simulink model "Ecotron"  (R2019b)
settings: Solver=FixedStepAuto  StartTime=0.0  StopTime=1  FixedStep=0.001  RelTol=1e-3  EnableMultiTasking=on
InitFcn:
  | EcoCoder_PreCheckLic();
libraries: CoderSF_BSW_Libs x228, SF_CanService_Libs x49, simulink x33, dspstat3 x6
(part 6 of 6)

== system Ecotron/Main /LongControl /ACC Control/Long PID/Acceleration ==
  speed : Inport
  Moving Average1 : dspstat3/Moving Average  Method=Sliding window  ForgettingFactorPort=off  SpecifyWindowLength=on  WindowLength=100  ForgettingFactor=0.9  SimulateUsing=Code generation
  Moving Average2 : dspstat3/Moving Average  Method=Sliding window  ForgettingFactorPort=off  SpecifyWindowLength=on  WindowLength=100  ForgettingFactor=0.9  SimulateUsing=Code generation
  Write Measurement : CoderSF_BSW_Libs/Calibration & Measurement/Write Measurement  variable_name=Golf_ACC  variable_value=0  variable_type=single  numD=1  unitStr=""  descStr=""
      settings: AttributesFormatString=type:%<variable_type> Dimensions:%<numD>  SourceProductName=EcoCoder Blocks
  Write Measurement1 : CoderSF_BSW_Libs/Calibration & Measurement/Write Measurement  variable_name=debug_Golf_speed  variable_value=0  variable_type=single  numD=1  unitStr=ms  descStr=""
      settings: AttributesFormatString=type:%<variable_type> Dimensions:%<numD>  SourceProductName=EcoCoder Blocks
  Write Measurement2 : CoderSF_BSW_Libs/Calibration & Measurement/Write Measurement  variable_name=debug_Golf_speed_movAvg  variable_value=0  variable_type=single  numD=1  unitStr=ms  descStr=""
      settings: AttributesFormatString=type:%<variable_type> Dimensions:%<numD>  SourceProductName=EcoCoder Blocks
  Write Measurement3 : CoderSF_BSW_Libs/Calibration & Measurement/Write Measurement  variable_name=debug_Golf_ACC  variable_value=0  variable_type=single  numD=1  unitStr=ms2  descStr=""
      settings: AttributesFormatString=type:%<variable_type> Dimensions:%<numD>  SourceProductName=EcoCoder Blocks
  basic derivative1 : Subsystem
  m/s^2 : Outport
  wires:
  Moving Average1/1 -> Write Measurement2/1, basic derivative1/1(In1)  "m/s"
  speed/1 -> Write Measurement1/1, Moving Average1/1
  basic derivative1/1(Out1) -> Write Measurement3/1, Moving Average2/1
  Moving Average2/1 -> Write Measurement/1, m/s^2/1  "m/s^2"

== system Ecotron/Main /LongControl /ACC Control/Long PID/Acceleration1 ==
  speed : Inport
  Moving Average1 : dspstat3/Moving Average  Method=Sliding window  ForgettingFactorPort=off  SpecifyWindowLength=on  WindowLength=200  ForgettingFactor=0.9  SimulateUsing=Code generation
  Moving Average2 : dspstat3/Moving Average  Method=Sliding window  ForgettingFactorPort=off  SpecifyWindowLength=on  WindowLength=200  ForgettingFactor=0.9  SimulateUsing=Code generation
  Write Measurement : CoderSF_BSW_Libs/Calibration & Measurement/Write Measurement  variable_name=Golf_ACC_200sample  variable_value=0  variable_type=single  numD=1  unitStr=""  descStr=""
      settings: AttributesFormatString=type:%<variable_type> Dimensions:%<numD>  SourceProductName=EcoCoder Blocks
  Write Measurement2 : CoderSF_BSW_Libs/Calibration & Measurement/Write Measurement  variable_name=debug_Golf_speed_movAvg150sample  variable_value=0  variable_type=single  numD=1  unitStr=ms  descStr=""
      settings: AttributesFormatString=type:%<variable_type> Dimensions:%<numD>  SourceProductName=EcoCoder Blocks
  Write Measurement3 : CoderSF_BSW_Libs/Calibration & Measurement/Write Measurement  variable_name=debug_Golf_ACC150sample  variable_value=0  variable_type=single  numD=1  unitStr=ms2  descStr=""
      settings: AttributesFormatString=type:%<variable_type> Dimensions:%<numD>  SourceProductName=EcoCoder Blocks
  basic derivative1 : Subsystem
  m/s^2 : Outport
  wires:
  Moving Average2/1 -> m/s^2/1, Write Measurement/1  "m/s^2"
  basic derivative1/1(Out1) -> Moving Average2/1, Write Measurement3/1
  speed/1 -> Moving Average1/1
  Moving Average1/1 -> basic derivative1/1(In1), Write Measurement2/1  "m/s"

== system Ecotron/Main /LongControl /ACC Control/Long PID/CascadedPID ==
  AccCMD : Inport
  m/s^2 : Inport  Port=2
  Motor torque : Inport  Port=3
  Gear : Inport  Port=4
  "Reset " : Inport  Port=5
  1-D Lookup Table : Lookup_n-D  NumberOfTableDimensions=1  BreakpointsForDimension1=[0:5]  Table=[0 118 194 291 390 516]  InternalRulePriority=Speed  RndMeth=Simplest  InputSameDT=on
  Multiply : Gain  Gain=0.01
  PID Controller : simulink/Continuous/PID Controller  Controller=PID  Form=Parallel  TimeDomain=Discrete-time  SampleTime=1/100  IntegratorMethod=Forward Euler  FilterMethod=Forward Euler  ControllerParametersSource=external  P=1  I=1  D=0  UseFilter=off  N=100  TunerSelectOption=Transfer Function Based (PID Tuner App)  InitialConditionSource=internal  InitialConditionForIntegrator=0  InitialConditionForFilter=0  DifferentiatorICPrevScaledInput=0  ExternalReset=either  TrackingMode=off  Kt=1  LimitOutput=on  UpperSaturationLimit=120  LowerSaturationLimit=0  LinearizeAsGain=on  AntiWindupMode=clamping  Kb=1  POutMin=[]  POutMax=[]  IOutMin=[]  IOutMax=[]  DOutMin=[]  DOutMax=[]  NOutMin=[]  NOutMax=[]  SumOutMin=[]  SumOutMax=[]  SaturationOutMin=[]  SaturationOutMax=[]  PParamMin=[]  PParamMax=[]  IParamMin=[]  IParamMax=[]  DParamMin=[]  DParamMax=[]  NParamMin=[]  NParamMax=[]  KbParamMin=[]  KbParamMax=[]  KtParamMin=[]  KtParamMax=[]  KbOutMin=[]  KbOutMax=[]  KtOutMin=[]  KtOutMax=[]  IntegratorOutMin=[]  IntegratorOutMax=[]  FilterOutMin=[]  FilterOutMax=[]  SumI1OutMin=[]  SumI1OutMax=[]  SumI2OutMin=[]  SumI2OutMax=[]  SumI3OutMin=[]  SumI3OutMax=[]  SumI4OutMin=[]  SumI4OutMax=[]  SumDOutMin=[]  SumDOutMax=[]  DifferentiatorOutMin=[]  DifferentiatorOutMax=[]  FilterDiffOutCoefMin=[]  FilterDiffOutCoefMax=[]  ReciprocalOutMin=[]  ReciprocalOutMax=[]  SumDenOutMin=[]  SumDenOutMax=[]  SumNumOutMin=[]  SumNumOutMax=[]  DivideOutMin=[]  DivideOutMax=[]  IntegratorContinuousStateAttributes=''  IntegratorStateMustResolveToSignalObject=off  IntegratorRTWStateStorageClass=Auto  FilterContinuousStateAttributes=''  FilterStateMustResolveToSignalObject=off  FilterRTWStateStorageClass=Auto  ParallelPVariant=ExternalParameters  IdealPVariant=Disabled  IVariant=ExternalParameters  DVariant=ExternalParameters  IntegratorVariant=Discrete  SatVariant=Enabled  AWVariant=DiscClampingParallel  PCopyVariant=Disabled  TRVariant=Disabled  FdbkBlocksVariant=Forward  IdealPFdbkVariant=Disabled  SatFdbkVariant=Disabled  DerivativeFilterVariant=Differentiator  NVariant=Passthrough  NCopyVariant=Disabled_SignalSpec  FilterICVariant=InternalICsDifferentiator  IntegratorICVariant=InternalICs  ExternalResetVariant=ExternalReset  TRSumVariant=Passthrough  SumFdbkVariant=Disabled  SumVariant=Sum_PID
  PID Controller1 : simulink/Continuous/PID Controller  Controller=PID  Form=Parallel  TimeDomain=Discrete-time  SampleTime=1/100  IntegratorMethod=Forward Euler  FilterMethod=Forward Euler  ControllerParametersSource=external  P=1  I=1  D=0  UseFilter=off  N=100  TunerSelectOption=Transfer Function Based (PID Tuner App)  InitialConditionSource=internal  InitialConditionForIntegrator=0  InitialConditionForFilter=0  DifferentiatorICPrevScaledInput=0  ExternalReset=either  TrackingMode=off  Kt=1  LimitOutput=on  UpperSaturationLimit=50  LowerSaturationLimit=0  LinearizeAsGain=on  AntiWindupMode=clamping  Kb=1  POutMin=[]  POutMax=[]  IOutMin=[]  IOutMax=[]  DOutMin=[]  DOutMax=[]  NOutMin=[]  NOutMax=[]  SumOutMin=[]  SumOutMax=[]  SaturationOutMin=[]  SaturationOutMax=[]  PParamMin=[]  PParamMax=[]  IParamMin=[]  IParamMax=[]  DParamMin=[]  DParamMax=[]  NParamMin=[]  NParamMax=[]  KbParamMin=[]  KbParamMax=[]  KtParamMin=[]  KtParamMax=[]  KbOutMin=[]  KbOutMax=[]  KtOutMin=[]  KtOutMax=[]  IntegratorOutMin=[]  IntegratorOutMax=[]  FilterOutMin=[]  FilterOutMax=[]  SumI1OutMin=[]  SumI1OutMax=[]  SumI2OutMin=[]  SumI2OutMax=[]  SumI3OutMin=[]  SumI3OutMax=[]  SumI4OutMin=[]  SumI4OutMax=[]  SumDOutMin=[]  SumDOutMax=[]  DifferentiatorOutMin=[]  DifferentiatorOutMax=[]  FilterDiffOutCoefMin=[]  FilterDiffOutCoefMax=[]  ReciprocalOutMin=[]  ReciprocalOutMax=[]  SumDenOutMin=[]  SumDenOutMax=[]  SumNumOutMin=[]  SumNumOutMax=[]  DivideOutMin=[]  DivideOutMax=[]  IntegratorContinuousStateAttributes=''  IntegratorStateMustResolveToSignalObject=off  IntegratorRTWStateStorageClass=Auto  FilterContinuousStateAttributes=''  FilterStateMustResolveToSignalObject=off  FilterRTWStateStorageClass=Auto  ParallelPVariant=ExternalParameters  IdealPVariant=Disabled  IVariant=ExternalParameters  DVariant=ExternalParameters  IntegratorVariant=Discrete  SatVariant=Enabled  AWVariant=DiscClampingParallel  PCopyVariant=Disabled  TRVariant=Disabled  FdbkBlocksVariant=Forward  IdealPFdbkVariant=Disabled  SatFdbkVariant=Disabled  DerivativeFilterVariant=Differentiator  NVariant=Passthrough  NCopyVariant=Disabled_SignalSpec  FilterICVariant=InternalICsDifferentiator  IntegratorICVariant=InternalICs  ExternalResetVariant=ExternalReset  TRSumVariant=Passthrough  SumFdbkVariant=Disabled  SumVariant=Sum_PID
  Product : Product
  Product1 : Product
  Read Calibration : CoderSF_BSW_Libs/Calibration & Measurement/Read Calibration  variable_name=Torque_PID_P  variable_value=0.15  variable_type=single  variable_min=[]  variable_max=[]  unitStr=""  descStr=""
      settings: AttributesFormatString=value:%<variable_value> type:%<variable_type> max:%<variable_max> Min:%<variable_min>  SourceProductName=EcoCoder Blocks
  Read Calibration1 : CoderSF_BSW_Libs/Calibration & Measurement/Read Calibration  variable_name=Torque_PID_I  variable_value=0.5  variable_type=single  variable_min=[]  variable_max=[]  unitStr=""  descStr=""
      settings: AttributesFormatString=value:%<variable_value> type:%<variable_type> max:%<variable_max> Min:%<variable_min>  SourceProductName=EcoCoder Blocks
  Read Calibration2 : CoderSF_BSW_Libs/Calibration & Measurement/Read Calibration  variable_name=Torque_PID_D  variable_value=0  variable_type=single  variable_min=[]  variable_max=[]  unitStr=""  descStr=""
      settings: AttributesFormatString=value:%<variable_value> type:%<variable_type> max:%<variable_max> Min:%<variable_min>  SourceProductName=EcoCoder Blocks
  Read Calibration3 : CoderSF_BSW_Libs/Calibration & Measurement/Read Calibration  variable_name=ACC_PID_P  variable_value=0.1  variable_type=single  variable_min=[]  variable_max=[]  unitStr=""  descStr=""
      settings: AttributesFormatString=value:%<variable_value> type:%<variable_type> max:%<variable_max> Min:%<variable_min>  SourceProductName=EcoCoder Blocks
  Read Calibration4 : CoderSF_BSW_Libs/Calibration & Measurement/Read Calibration  variable_name=ACC_PID_I  variable_value=0.4  variable_type=single  variable_min=[]  variable_max=[]  unitStr=""  descStr=""
      settings: AttributesFormatString=value:%<variable_value> type:%<variable_type> max:%<variable_max> Min:%<variable_min>  SourceProductName=EcoCoder Blocks
  Read Calibration5 : CoderSF_BSW_Libs/Calibration & Measurement/Read Calibration  variable_name=ACC_PID_D  variable_value=0  variable_type=single  variable_min=[]  variable_max=[]  unitStr=""  descStr=""
      settings: AttributesFormatString=value:%<variable_value> type:%<variable_type> max:%<variable_max> Min:%<variable_min>  SourceProductName=EcoCoder Blocks
  Subtract : Sum  Inputs=+-
  Subtract1 : Sum  Inputs=+-
  Write Measurement : CoderSF_BSW_Libs/Calibration & Measurement/Write Measurement  variable_name=Motor_requested_Torque  variable_value=0  variable_type=single  numD=1  unitStr=""  descStr=""
      settings: AttributesFormatString=type:%<variable_type> Dimensions:%<numD>  SourceProductName=EcoCoder Blocks
  Gas : Outport
  wires:
  AccCMD/1 -> Subtract/1
  m/s^2/1 -> Subtract/2
  Subtract/1 -> PID Controller/1
  Read Calibration/1 -> PID Controller1/2
  Read Calibration1/1 -> PID Controller1/3
  Read Calibration2/1 -> PID Controller1/4
  Gear/1 -> 1-D Lookup Table/1
  Read Calibration3/1 -> Product/1
  1-D Lookup Table/1 -> Product1/1, Product/2
  Read Calibration4/1 -> Product1/2
  Product/1 -> PID Controller/2
  Product1/1 -> PID Controller/3
  Read Calibration5/1 -> PID Controller/4
  Subtract1/1 -> PID Controller1/1
  PID Controller/1 -> Write Measurement/1, Subtract1/1  "Requested Torque"
  Motor torque/1 -> Subtract1/2
  PID Controller1/1 -> Multiply/1
  Multiply/1 -> Gas/1
  "Reset "/1 -> PID Controller1/5, PID Controller/5

== system Ecotron/Main /LongControl /ACC Control/Long PID/Level converter ==
  Pi in : Inport
  StopMode : Inport  Port=2
  Constant : Constant  Value=50  OutDataTypeStr=single
  Constant1 : Constant  Value=0  OutDataTypeStr=single
  Gain : Gain  Gain=-1
  Gain2 : Gain  Gain=120
  Gain4 : Gain  Gain=100
  Saturation : Saturate  UpperLimit=1  LowerLimit=0
  Saturation1 : Saturate  UpperLimit=1  LowerLimit=0
  Switch : Switch  Criteria=u2 > Threshold
  Switch1 : Switch  Criteria=u2 > Threshold
  Gas : Outport
  Brake : Outport  Port=2
  wires:
  Pi in/1 -> Gain/1, Saturation/1
  Saturation/1 -> Gain4/1  "gas"
  Gain/1 -> Saturation1/1
  StopMode/1 -> Switch1/2, Switch/2
  Saturation1/1 -> Gain2/1  "brake"
  Constant/1 -> Switch/1
  Constant1/1 -> Switch1/1
  Switch1/1 -> Gas/1
  Switch/1 -> Brake/1
  Gain2/1 -> Switch/3
  Gain4/1 -> Switch1/3

== system Ecotron/Main /LongControl /ACC Control/Fcalculator /Acceleration1/basic derivative1 ==
  In1 : Inport
  Constant : Constant  Value=0.001  OutDataTypeStr=single
  Divide : Product  Inputs=*/
  Subtract : Sum  Inputs=+-
  Unit Delay : UnitDelay  SampleTime=-1  HasFrameUpgradeWarning=on
  Out1 : Outport
  wires:
  Unit Delay/1 -> Subtract/2
  Subtract/1 -> Divide/1
  Constant/1 -> Divide/2
  Divide/1 -> Out1/1
  In1/1 -> Subtract/1, Unit Delay/1

== system Ecotron/Main /LongControl /ACC Control/Long PID/Acceleration/basic derivative1 ==
  In1 : Inport
  Constant : Constant  Value=0.001  OutDataTypeStr=single
  Divide : Product  Inputs=*/
  Subtract : Sum  Inputs=+-
  Unit Delay : UnitDelay  SampleTime=-1  HasFrameUpgradeWarning=on
  Out1 : Outport
  wires:
  In1/1 -> Unit Delay/1, Subtract/1
  Divide/1 -> Out1/1
  Constant/1 -> Divide/2
  Subtract/1 -> Divide/1
  Unit Delay/1 -> Subtract/2

== system Ecotron/Main /LongControl /ACC Control/Long PID/Acceleration1/basic derivative1 ==
  In1 : Inport
  Constant : Constant  Value=0.001  OutDataTypeStr=single
  Divide : Product  Inputs=*/
  Subtract : Sum  Inputs=+-
  Unit Delay : UnitDelay  SampleTime=-1  HasFrameUpgradeWarning=on
  Out1 : Outport
  wires:
  Unit Delay/1 -> Subtract/2
  Subtract/1 -> Divide/1
  Constant/1 -> Divide/2
  Divide/1 -> Out1/1
  In1/1 -> Subtract/1, Unit Delay/1

== stateflow chart Ecotron/Main /Gear/Gear_Control/Chart1 ==
  note: 1-Park
      | 2-R
      | 3-N
      | 4-D
  state high
    entry:
    PtoNTrigger=1;
    cnt = cnt + 1;
  state low
    entry:
    PtoNTrigger=0;
  state high1
    entry:
    PtoDTrigger=1;
    cnt = cnt + 1;
  state low1
    entry:
    PtoDTrigger=0;
  state init
    entry:
    cnt=0;
    PtoNTrigger = 0;
    PtoDTrigger=0;
    RtoNTrigger=0;
    NtoRTrigger=0;
    NtoDTrigger=0;
    DtoNTrigger=0;
  state high2
    entry:
    RtoNTrigger=1;
    cnt = cnt + 1;
  state low2
    entry:
    RtoNTrigger=0;
  state high3
    entry:
    NtoRTrigger=1;
    cnt = cnt + 1;
  state low3
    entry:
    NtoRTrigger=0;
  state high4
    entry:
    NtoDTrigger=1;
    cnt = cnt + 1;
  state low4
    entry:
    NtoDTrigger=0;
  state high5
    entry:
    DtoNTrigger=1;
    cnt = cnt + 1;
  state low5
    entry:
    DtoNTrigger=0;
  (junction 81) -> init : after(delay,msec)
  (junction 95) -> high [order 3] : [CurrentGear==1&&(SetGear==3||SetGear==2)]
  low -> high [order 2] : after(interval,msec)
  high -> low : after(interval2,msec)
  low -> (junction 81) [order 1] : [msglimit<=cnt]
  (junction 95) -> high1 [order 2] : [CurrentGear==1&&SetGear==4]
  (default) -> init
  low1 -> high1 [order 2] : after(interval,msec)
  high1 -> low1 : after(interval2,msec)
  low1 -> (junction 81) [order 1] : [msglimit<=cnt]
  low5 -> (junction 81) [order 1] : [msglimit<=cnt]
  (junction 95) -> high2 [order 4] : [CurrentGear==2&&(SetGear==3||SetGear==4)]
  low4 -> (junction 81) [order 1] : [msglimit<=cnt]
  low2 -> (junction 81) [order 1] : [msglimit<=cnt]
  low3 -> (junction 81) [order 1] : [msglimit<=cnt]
  init -> (junction 95) : [Available==1&&SetGear~=CurrentGear&&SetGear~=1&&ENABLE==1]
  (junction 95) -> high3 [order 1] : [CurrentGear==3&&SetGear==2]
  (junction 95) -> high4 [order 5] : [CurrentGear==3&&SetGear==4]
  (junction 95) -> high5 [order 6] : [CurrentGear==4&&(SetGear==2||SetGear==3)]
  low2 -> high2 [order 2] : after(interval,msec)
  high2 -> low2 : after(interval2,msec)
  low3 -> high3 [order 2] : after(interval,msec)
  high3 -> low3 : after(interval2,msec)
  low4 -> high4 [order 2] : after(interval,msec)
  high4 -> low4 : after(interval2,msec)
  low5 -> high5 [order 2] : after(interval,msec)
  high5 -> low5 : after(interval2,msec)
  data: cnt output; SetGear input uint8; CurrentGear input; Available input; PtoNTrigger output; interval input; msglimit input; PtoDTrigger output; DtoNTrigger output; NtoDTrigger output; NtoRTrigger output; RtoNTrigger output; interval2 input; delay input; ENABLE input

== stateflow chart Ecotron/Main /LateralControl/Chart ==
  state Otonom
    entry:
    EPAS_mode = 0; %angle mode
    during:
    EPAS_SteeringPosCMD = Set_SteeringPos;
    state Fast
      during:
      state up
        en:
        EPAS_Speedlimit = EPAS_Speedlimit + 1
      up -> (junction 93) : after(1,msec)
      (junction 93) -> (junction 95) [order 2]
      (junction 93) -> up [order 1] : [EPAS_Speedlimit<MaxEPASSpeed]
    state Slow
      entry:
      EPAS_Speedlimit = 50;
    (default) -> Slow
    Slow -> Fast : [Vehicle_Speed>3]
  state set
    entry:
    Epas_ECU_reset =true;
  state mod1
    entry:
    EPAS_mode = 1;
  state reset
    entry:
    Epas_ECU_reset = false;
  state Manual
    entry:
    EPAS_mode = 2; %free mode
    EPAS_SteeringPosCMD = 0;
    EPAS_Speedlimit = 50;
  (junction 49) -> Manual [order 2] : [AutonomyEnable==0]
  (default) -> Manual
  Manual -> mod1 : [AutonomyEnable==1]
  mod1 -> set [order 1] : after(10,msec)
  set -> reset : after(10,msec)
  reset -> (junction 49) : after(30,msec)
  (junction 49) -> Otonom [order 1] : [EPAS_intervention == 0]
  mod1 -> Manual [order 2] : [AutonomyEnable==0]
  Otonom -> Manual : [AutonomyEnable==0]
  data: AutonomyEnable input; EPAS_mode output uint8; EPAS_SteeringPosCMD output; EPAS_Speedlimit output; Vehicle_Speed input; Epas_ECU_reset output; EPAS_intervention input; MaxEPASSpeed input; Set_SteeringPos input

== stateflow chart Ecotron/Main /LongControl /Chart ==
  state PC
    during:
    Throttle_out = PC_Throttle;
    Brake_out = PC_Brake;
  state Manual
    entry:
    AutonomyEnable;
    LongMode;
    PC_Throttle;
    PC_Brake;
    Acc_Throttle;
    Acc_Brake;
    Throttle_out = 0;
    Brake_out = 0;
  state PC_Acc
    during:
    Throttle_out = Acc_Throttle;
    Brake_out = Acc_Brake;
  (default) -> Manual
  PC -> (junction 30) : [AutonomyEnable==0]
  (junction 3) -> PC [order 1] : [LongMode==1]
  Manual -> (junction 3) : [AutonomyEnable==1]
  (junction 3) -> PC_Acc [order 2] : [LongMode==0]
  PC_Acc -> (junction 30) : [AutonomyEnable==0]
  (junction 30) -> Manual
  data: AutonomyEnable input; LongMode input; PC_Brake input; PC_Throttle input; Brake_out output; Throttle_out output; Acc_Throttle input single; Acc_Brake input single

== stateflow chart Ecotron/Subsystem4/PC/Chart ==
  state Hazard
    entry:
    output = 3;
  state init
    entry:
    output = 0;
  state left
    entry:
    output = 1;
  state right
    entry:
    output = 2;
  Hazard -> left [order 2] : [left==1]
  (default) -> init
  Hazard -> init [order 1] : [Hazard==0]
  init -> left [order 1] : [left==1]
  left -> init [order 1] : [left==0]
  init -> Hazard [order 3] : [Hazard==1]
  Hazard -> right [order 3] : [right==1]
  right -> init [order 1] : [right==0]
  init -> right [order 2] : [right==1]
  left -> right [order 2] : [right==1]
  right -> left [order 2] : [left==1]
  data: left input; right input; output output; Hazard input

== stateflow chart Ecotron/Main /LongControl /Brake Calib logic/Chart ==
  state SetCalibCMD
    entry:
    Calib_CMD = true;
  state init
    entry:
    Calib_CMD = false;
  (default) -> init
  init -> SetCalibCMD : [BrakePedalPos < 3 && isMotorRunning == true && BBW_CalibrationErr == true && speed < 0.05 ]
  SetCalibCMD -> init [order 2] : [BBW_CalibrationErr == false && BBW_OnCalibration == false]
  SetCalibCMD -> SetCalibCMD [order 1] : [BBW_OnCalibration == true]
  data: isMotorRunning input; BrakePedalPos input; BBW_OnCalibration input; BBW_CalibrationErr input; Calib_CMD output boolean; speed input

== stateflow chart Ecotron/Main /Mode Select/Chart ==
  state Manual
    entry:
    Mode = false;
  state Autonomous
    entry:
    Mode = true;
  (default) -> Manual
  Manual -> Autonomous : [AutonomyEnable > 0 && AutonomyDisable~=1&& Errors == 0&&HandBrake>0.5]
  Autonomous -> Manual : [Errors > 0||AutonomyDisable==1]
  data: Mode output boolean; Errors input boolean; AutonomyEnable input boolean; AutonomyDisable input; HandBrake input

== stateflow chart Ecotron/Main /Gear/Gear_Control/Chart ==
  state init
    entry:
    Parktrigger = false;
  state trigger
    entry:
    Parktrigger = true;
  (default) -> init
  init -> trigger : [SetGear~=CurrentGear&&SetGear==1&&ENABLE==1]
  trigger -> init : after(250,msec)
  data: CurrentGear input; SetGear input; Parktrigger output boolean; ENABLE input

== stateflow chart Ecotron/Main /LongControl /ACC Control/StopModeDesicion/Chart1 ==
  state Move
    entry:
    Stopmode = false
  state StopMode
    entry:
    Stopmode = true
  (default) -> StopMode
  StopMode -> Move : [Acc > 0.05 && (Gear == 2 || Gear == 4)]
  Move -> StopMode : [(Speed < 0.1 && Acc < -0.05)||(Gear ==1)||mode==0]
  data: Stopmode output boolean; Acc input; Gear input; mode input; Speed input

== stateflow chart Ecotron/Subsystem4/Button cntrl /Chart ==
  state HazardON
    state Set
      entry:
      Output=1;
    state Reset
      entry:
      Output = 0;
    (default) -> HazardON.Set
    HazardON.Set -> HazardON.Reset : after(50,msec)
    (junction 32) -> HazardON.Set : [HazardState==0]
    HazardON.Reset -> (junction 32) : after(500,msec)
  state init
    entry:
    Output = 0;
  state HazardOFF
    state Set
      entry:
      Output=1;
    state Reset
      entry:
      Output = 0;
    (default) -> HazardOFF.Set
    HazardOFF.Set -> HazardOFF.Reset : after(50,msec)
    (junction 22) -> HazardOFF.Set : [HazardState==1]
    HazardOFF.Reset -> (junction 22) : after(500,msec)
  (default) -> init
  init -> HazardON [order 1] : [SetHazard==1&& HazardState==0]
  HazardON -> init : [SetHazard==1&& HazardState==1]
  HazardOFF -> init : [SetHazard==0&& HazardState==0]
  init -> HazardOFF [order 2] : [SetHazard==0&& HazardState==1]
  data: SetHazard input; HazardState input; Output output

== stateflow chart Ecotron/Main /LongControl /ACC Control/Long PID/Chart ==
  state Brake
    entry:
    State=false;
  state Gas
    entry:
    State=true;
  (default) -> Brake
  Brake -> Gas : [duration(Acc > AccThreshold) > Duration || Acc > 2 *AccThreshold]
  Gas -> Brake : [duration(Acc < -AccThreshold)> Duration||StopMode==1||Acc < -2 *AccThreshold]
  data: StopMode input; Acc input; AccThreshold input; State output boolean; Duration input

== stateflow chart Ecotron/Main /PDS StartupShutdown/Chart ==
  state Startup
    state VLS128
      entry:
      Channel=3;
      Onoff=1;
      Msgtrigger=1;
      during:
      Msgtrigger=0;
    state LIDARS
      entry:
      Channel=1;
      Onoff=1;
      Msgtrigger=1;
      during:
      Msgtrigger=0;
    state Modem
      entry:
      Channel=4;
      Onoff=1;
      Msgtrigger=1;
      during:
      Msgtrigger=0;
    state GNSS
      entry:
      Channel=2;
      Onoff=1;
      Msgtrigger=1;
      during:
      Msgtrigger=0;
    state DBW
      entry:
      Channel=5;
      Onoff=1;
      Msgtrigger=1;
      exit:
      Msgtrigger=0;
    state Brake
      entry:
      Channel=7;
      Onoff=1;
      Msgtrigger=1;
      during:
      Msgtrigger=0;
    state EPAS
      entry:
      Channel=9;
      Onoff=1;
      Msgtrigger=1;
      during:
      Msgtrigger=0;
    (default) -> Startup.Modem
    Startup.Modem -> Startup.GNSS : after(200,msec)
    Startup.VLS128 -> Startup.LIDARS : after(500,msec)
    Startup.GNSS -> Startup.VLS128 : after(500,msec)
    Startup.LIDARS -> Startup.EPAS : after(500,msec)
    Startup.Brake -> Startup.DBW : after(500,msec)
    Startup.EPAS -> Startup.Brake : after(500,msec)
  state start
    entry:
    Channel=0;
    Onoff=0;
    Msgtrigger=0;
  state Shutdown
    state VLS128
      entry:
      Channel=3;
      Onoff=0;
      Msgtrigger=1;
      during:
      Msgtrigger=0;
    state LIDARS
      entry:
      Channel=1;
      Onoff=0;
      Msgtrigger=1;
      during:
      Msgtrigger=0;
    state Modem
      entry:
      Channel=4;
      Onoff=0;
      Msgtrigger=1;
      during:
      Msgtrigger=0;
    state GNSS
      entry:
      Channel=2;
      Onoff=0;
      Msgtrigger=1;
      during:
      Msgtrigger=0;
    state DBW
      entry:
      Channel=5;
      Onoff=0;
      Msgtrigger=1;
      exit:
      Msgtrigger=0;
    state Brake
      entry:
      Channel=7;
      Onoff=0;
      Msgtrigger=1;
      during:
      Msgtrigger=0;
    state EPAS
      entry:
      Channel=9;
      Onoff=0;
      Msgtrigger=1;
      during:
      Msgtrigger=0;
    (default) -> Shutdown.Modem
    Shutdown.Modem -> Shutdown.GNSS : after(200,msec)
    Shutdown.VLS128 -> Shutdown.LIDARS : after(200,msec)
    Shutdown.GNSS -> Shutdown.VLS128 : after(200,msec)
    Shutdown.LIDARS -> Shutdown.EPAS : after(200,msec)
    Shutdown.Brake -> Shutdown.DBW : after(200,msec)
    Shutdown.EPAS -> Shutdown.Brake : after(200,msec)
  (default) -> start
  Startup.DBW -> start
  start -> Startup [order 1] : [risingedge==1]
  start -> Shutdown [order 2] : [fallingedge==1]
  Shutdown.DBW -> start
  Shutdown -> Startup : [risingedge==1]
  Startup -> Shutdown : [fallingedge==1]
  data: risingedge input; fallingedge input; Channel output; Onoff output; Msgtrigger output

== stateflow chart Ecotron/Subsystem4/Button cntrl /Subsystem4/Chart ==
  state risingBuzz
    entry:
    Output = true;
  state NoBuzz
    entry:
    Output = false;
  state FallingBuzz
    entry:
    repeat = 0;
    state OFF
      entry:
      Output = false;
      repeat = repeat + 1;
    state ON
      entry:
      Output = true;
    (default) -> ON
    ON -> OFF : after(falling_duration,msec)
    OFF -> ON : [after(falling_offduration,msec)&&repeat < 3]
  (default) -> NoBuzz
  NoBuzz -> risingBuzz [order 1] : [risingedge > 0]
  risingBuzz -> FallingBuzz [order 2] : [fallingedge > 0]
  risingBuzz -> NoBuzz [order 1] : after(rising_duration,msec)
  FallingBuzz -> risingBuzz [order 2] : [risingedge > 0]
  FallingBuzz -> NoBuzz [order 1] : [repeat >= 3]
  NoBuzz -> FallingBuzz [order 2] : [fallingedge > 0]
  data: risingedge input; fallingedge input; rising_duration input; falling_duration input; Output output boolean; repeat local; falling_offduration input
